simulink model "controle_mpc"  (R2020b)
settings: Solver=ode4  StartTime=0.0  StopTime=30  FixedStep=h_plant  RelTol=1e-3
values from neighbouring files (symbols this model uses):
  A = [0 1; 0 0]    [controle_mpc_script.m]
  B = [0; 1]    [controle_mpc_script.m]
  C = [1 0]    [controle_mpc_script.m]
  Gamma = [h^2/2; h]    [controle_mpc_script.m]
  h = 1    [controle_mpc_script.m]
  h_plant = (1e-4)    (= 0.0001)    [controle_mpc_script.m]
  measure_noise_gain = 1    [controle_mpc_script.m]
  N = 20    [controle_mpc_script.m]
  n = length(Phi)    [controle_mpc_script.m]
  Phi = [1 h; 0 1]    [controle_mpc_script.m]
  Q0 = eye(n)    [controle_mpc_script.m]
  Q1 = eye(n)    [controle_mpc_script.m]
  Q2 = 1/10    (= 0.1)    [controle_mpc_script.m]
  sat_max = 10    [controle_mpc_script.m]
  sat_min = -10    [controle_mpc_script.m]
  UM = 100    [controle_mpc_script.m]
  Um = -100    [controle_mpc_script.m]
  wind_final_value = 0.2    [controle_mpc_script.m]
  wind_initial_value = 0    [controle_mpc_script.m]
  wind_steptime = 0    [controle_mpc_script.m]
  x0 = zeros(2, 1)    [controle_mpc_script.m]
  YM = 100    [controle_mpc_script.m]
  Ym = -100    [controle_mpc_script.m]
libraries: simulink x2, eeLuenbergerObserver x1
settings Model: Creator=Trevor  LastModifiedBy=lucas
settings SolverCC: AutoInsertRateTranBlk=on
settings DataIOCC: LimitDataPoints=on  SaveFormat=Array  ReturnWorkspaceOutputs=off
settings OptimizationCC: LifeSpan=inf
settings DebuggingCC: SFUnexpectedBacktrackingDiag=warning  SFNoUnconditionalDefaultTransitionDiag=warning  SFExecutionAtInitializationDiag=none  ArithmeticOperatorsInVariantConditions=warning
settings HardwareCC: ProdBitPerPointer=32  ProdBitPerSizeT=32  ProdBitPerPtrDiffT=32  ProdLargestAtomicFloat=None  ProdIntDivRoundTo=Undefined  ProdEndianess=Unspecified  ProdWordSize=32  ProdHWDeviceType=32-bit Generic
settings ModelReferenceCC: PropagateSignalLabelsOutOfModel=off
settings SFSimCC: SimUseLocalCustomCode=off  CustomCodeUndefinedFunction=UseInterfaceOnly
settings RTWCC: RTWUseLocalCustomCode=off
settings CodeAppCC: StateflowObjectComments=on
settings GRTTargetCC: TargetLangStandard=C89/C90 (ANSI)
settings ConfigComp: CovMetricSettings=dw  CovSaveCumulativeToWorkspaceVar=on  CovSaveSingleToWorkspaceVar=on  CovExternalEMLEnable=off

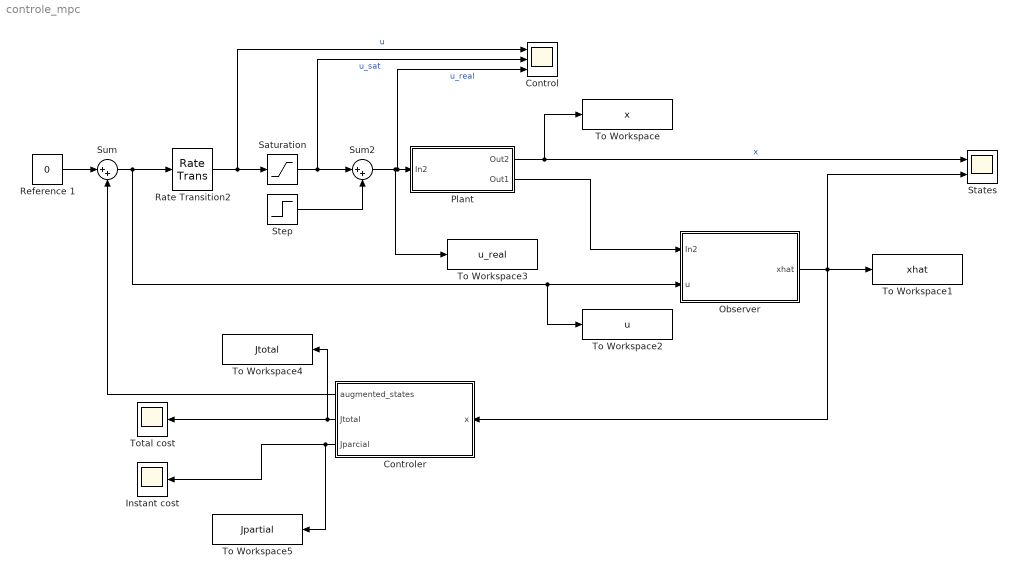
== system controle_mpc ==
  Control : Scope  NumInputPorts=3
  Controler : Subsystem
  Instant cost : Scope
  Observer : Subsystem
  Plant : Subsystem
  Rate Transition2 : RateTransition  Integrity=off  OutPortSampleTimeMultiple=0.01  OutPortSampleTime=h_plant
  Reference 1 : Constant  Value=0  SampleTime=h
  Saturation : Saturate  UpperLimit=sat_max  LowerLimit=sat_min
  States : Scope  NumInputPorts=2
  Step : Step  Time=wind_steptime  Before=wind_initial_value  After=wind_final_value  SampleTime=h_plant
  Sum : Sum  Inputs=|++
  Sum2 : Sum  Inputs=|++
  To Workspace : ToWorkspace  VariableName=x  SaveFormat=Timeseries  SampleTime=-1
  To Workspace1 : ToWorkspace  VariableName=xhat  SaveFormat=Timeseries  SampleTime=-1
  To Workspace2 : ToWorkspace  VariableName=u  SaveFormat=Timeseries  SampleTime=-1
  To Workspace3 : ToWorkspace  VariableName=u_real  SaveFormat=Timeseries  SampleTime=-1
  To Workspace4 : ToWorkspace  VariableName=Jtotal  SaveFormat=Timeseries  SampleTime=-1
  To Workspace5 : ToWorkspace  VariableName=Jpartial  SaveFormat=Timeseries  SampleTime=-1
  Total cost : Scope
  wires:
  Sum/1 -> To Workspace2/1, Observer/2(u), Rate Transition2/1
  Reference 1/1 -> Sum/1
  Plant/1(Out2) -> To Workspace/1, States/1  "x"
  Saturation/1 -> Sum2/1, Control/2  "u_sat"
  Rate Transition2/1 -> Saturation/1, Control/1  "u"
  Sum2/1 -> To Workspace3/1, Control/3, Plant/1(In2)  "u_real"
  Step/1 -> Sum2/2
  Observer/1(xhat) -> To Workspace1/1, States/2, Controler/1(x)
  Plant/2(Out1) -> Observer/1(In2)
  Controler/1(augmented_states) -> Sum/2
  Controler/2(Jtotal) -> To Workspace4/1, Total cost/1
  Controler/3(Jparcial) -> To Workspace5/1, Instant cost/1

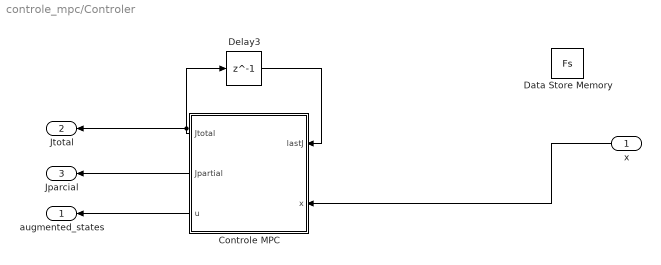
== system controle_mpc/Controler ==
  x : Inport
  Controle MPC : MATLAB Function  TreatAsAtomicUnit=on
  Data Store Memory : DataStoreMemory  DataStoreName=Fs  ReadBeforeWriteMsg=warning  WriteAfterWriteMsg=warning  WriteAfterReadMsg=warning  InitialValue=zeros(1,n,1,N)  VectorParams1D=off  ShowAdditionalParam=off  OutDataTypeStr=double
  Delay3 : Delay  DelayLength=1  SampleTime=h
  augmented_states : Outport
  Jtotal : Outport  Port=2
  Jparcial : Outport  Port=3
  wires:
  Controle MPC/1(Jtotal) -> Jtotal/1, Delay3/1
  x/1 -> Controle MPC/2(x)
  Controle MPC/2(Jpartial) -> Jparcial/1
  Delay3/1 -> Controle MPC/1(lastJ)
  Controle MPC/3(u) -> augmented_states/1

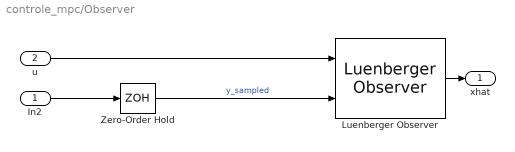
== system controle_mpc/Observer ==
  In2 : Inport
  u : Inport  Port=2
  Luenberger Observer : eeLuenbergerObserver/Luenberger Observer  StateSpaceType=Discrete-time  Ad=Phi  Bd=Gamma  Cd=C_discrete  Dd=D_discrete  A=1  B=1  C=1  D=1  ObserverDesign=Desired eigenvalues  Ld=1  DesiredEigenvalues=observer_eig  x0=x0_observer  Tsd=0.1  Ts=h
      settings: SourceProductBaseCode=PS
  Zero-Order Hold : ZeroOrderHold  SampleTime=h
  xhat : Outport
  wires:
  Zero-Order Hold/1 -> Luenberger Observer/2  "y_sampled"
  Luenberger Observer/1 -> xhat/1
  In2/1 -> Zero-Order Hold/1
  u/1 -> Luenberger Observer/1

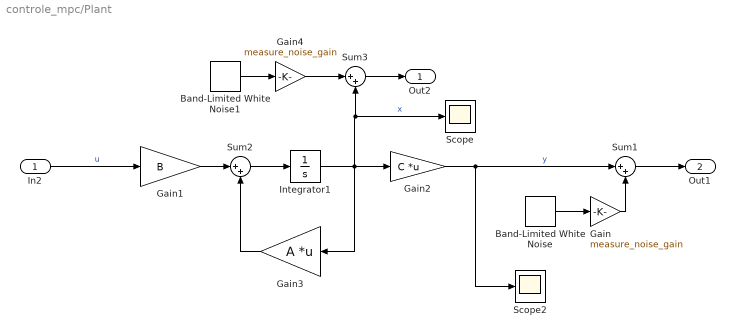
== system controle_mpc/Plant ==
  In2 : Inport
  Band-Limited White Noise : simulink/Sources/Band-Limited White Noise  Cov=[1e-6]  Ts=h  seed=[23341]
  Band-Limited White Noise1 : simulink/Sources/Band-Limited White Noise  Cov=[1e-6]  Ts=h  seed=[23341]
  Gain : Gain  Gain=measure_noise_gain
  Gain1 : Gain  Gain=B
  Gain2 : Gain  Gain=C  Multiplication=Matrix(K*u) (u vector)
  Gain3 : Gain  Gain=A  Multiplication=Matrix(K*u) (u vector)
  Gain4 : Gain  Gain=measure_noise_gain
  Integrator1 : Integrator  InitialCondition=x0
  Scope : Scope
  Scope2 : Scope
  Sum1 : Sum  Inputs=|++
  Sum2 : Sum  Inputs=|++
  Sum3 : Sum  Inputs=|++
  Out2 : Outport
  Out1 : Outport  Port=2
  wires:
  Gain3/1 -> Sum2/2
  Integrator1/1 -> Gain3/1, Sum3/2, Scope/1, Gain2/1  "x"
  Sum2/1 -> Integrator1/1
  Gain1/1 -> Sum2/1
  In2/1 -> Gain1/1  "u"
  Gain2/1 -> Sum1/1, Scope2/1  "y"
  Band-Limited White Noise/1 -> Gain/1
  Gain/1 -> Sum1/2
  Sum1/1 -> Out1/1
  Gain4/1 -> Sum3/1
  Band-Limited White Noise1/1 -> Gain4/1
  Sum3/1 -> Out2/1

== matlab function controle_mpc/Controler/Controle MPC ==
  settings: updateMethod=DISCRETE  sampleTime=h
  data: Jtotal output; Jpartial output; lastJ input; Q1 parameter; Q2 parameter; Q0 parameter; n parameter; Phi parameter; Gamma parameter; x input; N parameter; C parameter; Fs data_store_memory; u output; UM parameter; Um parameter; YM parameter; Ym parameter
function [Jtotal,Jpartial,u] = fcn(lastJ,Q1,Q2,Q0,n,Phi,Gamma,x,N,C,UM, Um, YM, Ym)
%#codegen

tStart = tic;

coder.extrinsic('quadprog');

U = zeros(N,1);
Gain = zeros(2,1);
Jpartial = 0;
Jtotal=0;
fval = 0;
z = zeros(N,1);

M0 = [Phi];
coder.varsize("Mu");
Mu = [Gamma, zeros(size(Gamma,1), N-1)];
Mu_aux = Mu;
Qtil =  kron(eye((N-1)*(n-1)), Q1);
Rbar = kron(eye(N*size(Gamma,2)), Q2);
Qbar = blkdiag(Qtil, Q0);
for i = 1:N-1
    M0 = [M0; Phi^(i+1)];
end
for i = 1:N-1
    Mu_aux = [Mu_aux(1)*Gamma, Mu_aux(:,1:length(Mu_aux)-1)];
    Mu = [Mu; Mu_aux];
end
Qxo = Q1 + M0'*Qbar*M0;
Qu = 2*Mu'*Qbar*Mu + Rbar;
Qxu = 2*M0'*Qbar*Mu;


% %Restrição na entrada
% G_entrada = [eye(N); -eye(N)];
% W_entrada = [UM*ones(N,1);  -Um*ones(N,1)];
% S_entrada = zeros(2*N,n);
% 
% %Restrição na saída(superior)
% G_ss_aux = [Gamma, zeros(n, N-1)]
% G_ss = [C*G_ss_aux]
% for i = 1:N-1
%     G_ss_aux = [Phi*G_ss_aux(1), G_ss_aux(:,1:length(G_ss_aux)-N)]
%     G_ss = [G_ss; C*G_ss_aux]
% end
% W_ss = [YM*ones(N,1)];
% S_si = [C*Phi];
% for i = 1:N-1
%     S_si = [S_si; C*Phi^(i+1)];
% end
% S_ss = -S_si;
% s = [S_entrada; S_ss];
% 
% 
% 
% 
% %Restrição na saída(inferior)
% G_si = -G_ss;
% W_si = [-Ym*ones(N,1)];
% 
% 
% %Parâmetros da função a restrição
% G_teste = [G_si;G_entrada];
% W_teste = [W_si;W_entrada];
% S_teste = [S_si;S_entrada];


[U , fval] = quadprog(2*Qu, 2*Qxu'*x);%, G_teste, W_teste + S_teste*x);
u = U(1,:);
Jpartial =  fval + x'*Qxo*x;
Jtotal = Jpartial+lastJ;

tEnd = toc(tStart);

% G1 = OutroH\OutroF;
% Gain = (evec*G1)';
% u = Gain'*x;
% z = -G1*x;
% Jpartial = 1/2*z'*OutroH*z+x'*OutroF'*z+x'*(Q1+M0'*Qbar*M0)*x;
% Jtotal = Jpartial+lastJ;
